simulink model "Selector"  (R2017a)
settings: Solver=VariableStepAuto  StartTime=0.0  StopTime=10.0  RelTol=1e-3
libraries: commrandsrc3 x1
settings Model: Creator=Arthur  LastModifiedBy=Arthur

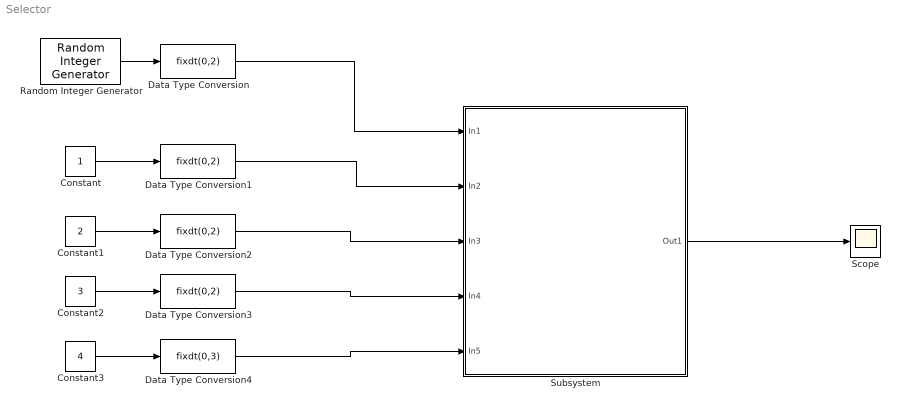
== system Selector ==
  Constant : Constant
  Constant1 : Constant  Value=2
  Constant2 : Constant  Value=3
  Constant3 : Constant  Value=4
  Data Type Conversion : DataTypeConversion  OutMin=0  OutMax=3  OutDataTypeStr=fixdt(0,2)
  Data Type Conversion1 : DataTypeConversion  OutMin=1  OutMax=1  OutDataTypeStr=fixdt(0,2)
  Data Type Conversion2 : DataTypeConversion  OutMin=2  OutMax=2  OutDataTypeStr=fixdt(0,2)
  Data Type Conversion3 : DataTypeConversion  OutMin=3  OutMax=3  OutDataTypeStr=fixdt(0,2)
  Data Type Conversion4 : DataTypeConversion  OutMin=4  OutMax=4  OutDataTypeStr=fixdt(0,3)
  Random Integer Generator : commrandsrc3/Random Integer Generator  SetSize=4  SeedSource=Auto  Seed=0  SampleTime=1  SamplesPerFrame=1  OutputDataType=double  SimulateUsing=Interpreted execution
  Scope : Scope
  Subsystem : Subsystem
  wires:
  Random Integer Generator/1 -> Data Type Conversion/1
  Constant3/1 -> Data Type Conversion4/1
  Constant2/1 -> Data Type Conversion3/1
  Constant1/1 -> Data Type Conversion2/1
  Constant/1 -> Data Type Conversion1/1
  Data Type Conversion/1 -> Subsystem/1(In1)
  Data Type Conversion1/1 -> Subsystem/2(In2)
  Data Type Conversion2/1 -> Subsystem/3(In3)
  Data Type Conversion3/1 -> Subsystem/4(In4)
  Data Type Conversion4/1 -> Subsystem/5(In5)
  Subsystem/1(Out1) -> Scope/1

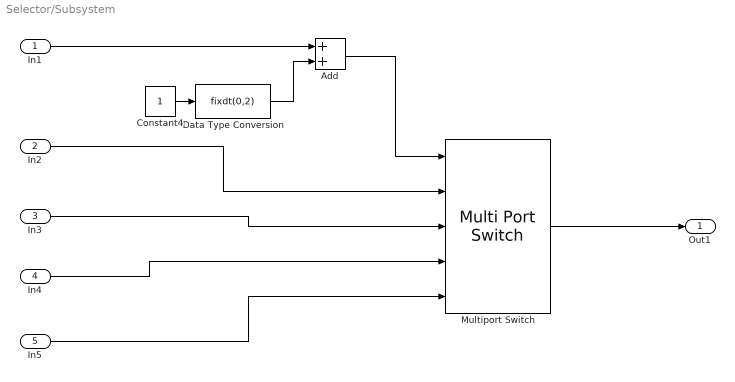
== system Selector/Subsystem ==
  In1 : Inport
  In2 : Inport  Port=2
  In3 : Inport  Port=3
  In4 : Inport  Port=4
  In5 : Inport  Port=5
  Add : Sum  OutMin=1  OutMax=4  OutDataTypeStr=fixdt(0,3)
  Constant4 : Constant  OutMin=1  OutMax=1  OutDataTypeStr=fixdt(0,2)
  Data Type Conversion : DataTypeConversion  OutMin=1  OutMax=1  OutDataTypeStr=fixdt(0,2)
  Multiport Switch : MultiPortSwitch  Inputs=4  DataPortIndices={1,2,3,4}  OutMin=1  OutMax=4  OutDataTypeStr=fixdt(0,3)
  Out1 : Outport
  wires:
  In3/1 -> Multiport Switch/3
  Add/1 -> Multiport Switch/1
  In5/1 -> Multiport Switch/5
  In1/1 -> Add/1
  In2/1 -> Multiport Switch/2
  Multiport Switch/1 -> Out1/1
  Data Type Conversion/1 -> Add/2
  Constant4/1 -> Data Type Conversion/1
  In4/1 -> Multiport Switch/4
